simulink model "test_script"  (R2019b)
settings: Solver=VariableStepAuto  StartTime=0.0  StopTime=10.0  RelTol=1e-3
settings Model: Creator=FX622208  LastModifiedBy=FX622208

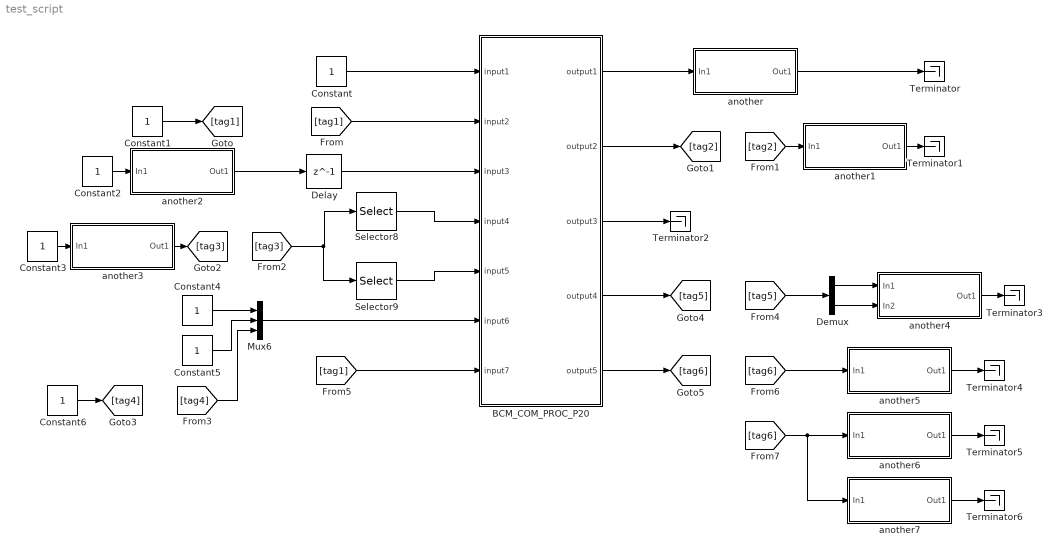
== system test_script ==
  BCM_COM_PROC_P20 : Subsystem
  Constant{,1..6} (7 alike) : Constant
  Delay : Delay  DelayLength=1  InitialCondition=0
  Demux : Demux  Outputs=2
  Mux6 : Mux  Inputs=3
  Selector8 : Selector  InputPortWidth=4  IndexOptions=Index vector (dialog)  Indices=[1 2]  OutputSizes=1
  Selector9 : Selector  InputPortWidth=4  IndexOptions=Index vector (dialog)  Indices=[3 4]  OutputSizes=1
  Terminator{,1..6} (7 alike) : Terminator
  another : Subsystem
  another1 : Subsystem
  another2 : Subsystem
  another3 : Subsystem
  another4 : Subsystem
  another5 : Subsystem
  another6 : Subsystem
  another7 : Subsystem
  wires:
  Constant/1 -> BCM_COM_PROC_P20/1(input1)
  BCM_COM_PROC_P20/1(output1) -> another/1(In1)
  [tag1] -> BCM_COM_PROC_P20/2(input2)
  Constant1/1 -> [tag1]
  BCM_COM_PROC_P20/2(output2) -> [tag2]
  [tag2] -> another1/1(In1)
  another/1(Out1) -> Terminator/1
  another1/1(Out1) -> Terminator1/1
  Constant2/1 -> another2/1(In1)
  another2/1(Out1) -> Delay/1
  Delay/1 -> BCM_COM_PROC_P20/3(input3)
  BCM_COM_PROC_P20/3(output3) -> Terminator2/1
  Selector8/1 -> BCM_COM_PROC_P20/4(input4)
  Selector9/1 -> BCM_COM_PROC_P20/5(input5)
  [tag3] -> Selector9/1, Selector8/1
  another3/1(Out1) -> [tag3]
  Constant3/1 -> another3/1(In1)
  Mux6/1 -> BCM_COM_PROC_P20/6(input6)
  Constant4/1 -> Mux6/1
  Constant5/1 -> Mux6/2
  [tag4] -> Mux6/3
  Constant6/1 -> [tag4]
  BCM_COM_PROC_P20/4(output4) -> [tag5]
  [tag5] -> Demux/1
  Demux/1 -> another4/1(In1)
  Demux/2 -> another4/2(In2)
  another4/1(Out1) -> Terminator3/1
  [tag1] -> BCM_COM_PROC_P20/7(input7)
  BCM_COM_PROC_P20/5(output5) -> [tag6]
  [tag6] -> another5/1(In1)
  another5/1(Out1) -> Terminator4/1
  another6/1(Out1) -> Terminator5/1
  [tag6] -> another7/1(In1), another6/1(In1)
  another7/1(Out1) -> Terminator6/1

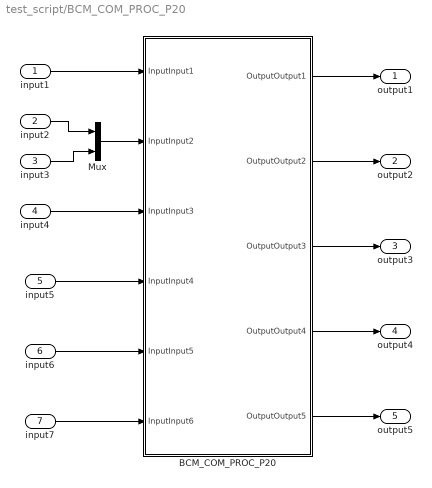
== system test_script/BCM_COM_PROC_P20 ==
  input1 : Inport
  input2 : Inport  Port=2
  input3 : Inport  Port=3
  input4 : Inport  Port=4
  input5 : Inport  Port=5
  input6 : Inport  Port=6
  input7 : Inport  Port=7
  BCM_COM_PROC_P20 : Subsystem
  Mux : Mux  Inputs=2
  output1 : Outport
  output2 : Outport  Port=2
  output3 : Outport  Port=3
  output4 : Outport  Port=4
  output5 : Outport  Port=5
  wires:
  input1/1 -> BCM_COM_PROC_P20/1(InputInput1)
  BCM_COM_PROC_P20/1(OutputOutput1) -> output1/1
  BCM_COM_PROC_P20/3(OutputOutput3) -> output3/1
  BCM_COM_PROC_P20/2(OutputOutput2) -> output2/1
  input2/1 -> Mux/1
  input3/1 -> Mux/2
  Mux/1 -> BCM_COM_PROC_P20/2(InputInput2)
  input4/1 -> BCM_COM_PROC_P20/3(InputInput3)
  BCM_COM_PROC_P20/4(OutputOutput4) -> output4/1
  input5/1 -> BCM_COM_PROC_P20/4(InputInput4)
  input6/1 -> BCM_COM_PROC_P20/5(InputInput5)
  input7/1 -> BCM_COM_PROC_P20/6(InputInput6)
  BCM_COM_PROC_P20/5(OutputOutput5) -> output5/1

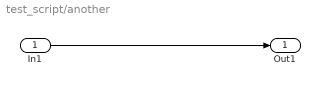
== system test_script/another ==
  In1 : Inport
  Out1 : Outport
  wires:
  In1/1 -> Out1/1

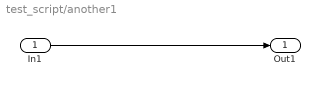
== system test_script/another1 ==
  In1 : Inport
  Out1 : Outport
  wires:
  In1/1 -> Out1/1

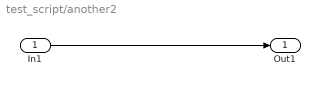
== system test_script/another2 ==
  In1 : Inport
  Out1 : Outport
  wires:
  In1/1 -> Out1/1

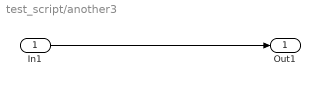
== system test_script/another3 ==
  In1 : Inport
  Out1 : Outport
  wires:
  In1/1 -> Out1/1

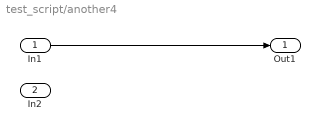
== system test_script/another4 ==
  In1 : Inport
  In2 : Inport  Port=2
  Out1 : Outport
  wires:
  In1/1 -> Out1/1

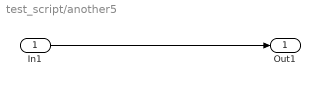
== system test_script/another5 ==
  In1 : Inport
  Out1 : Outport
  wires:
  In1/1 -> Out1/1

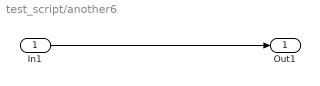
== system test_script/another6 ==
  In1 : Inport
  Out1 : Outport
  wires:
  In1/1 -> Out1/1

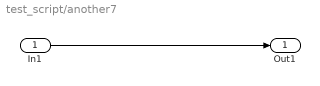
== system test_script/another7 ==
  In1 : Inport
  Out1 : Outport
  wires:
  In1/1 -> Out1/1

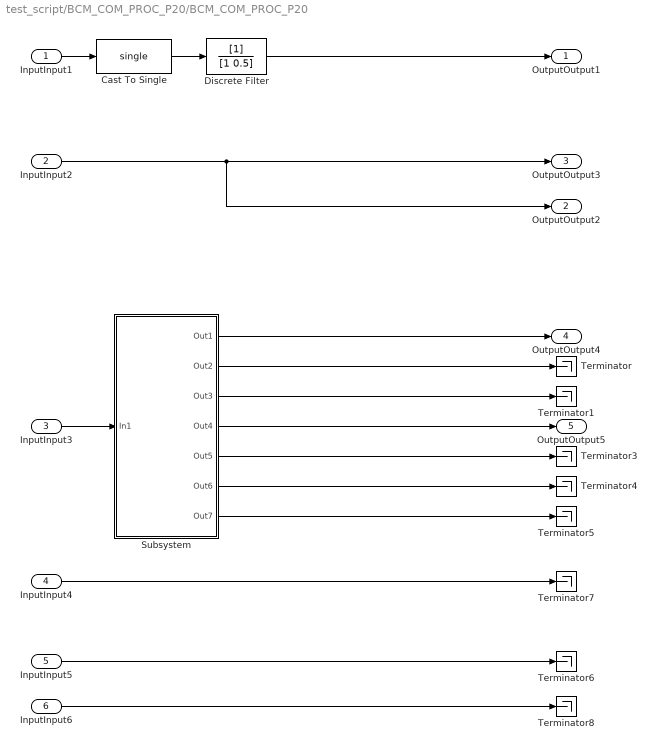
== system test_script/BCM_COM_PROC_P20/BCM_COM_PROC_P20 ==
  InputInput1 : Inport
  InputInput2 : Inport  Port=2
  InputInput3 : Inport  Port=3
  InputInput4 : Inport  Port=4
  InputInput5 : Inport  Port=5
  InputInput6 : Inport  Port=6
  Cast To Single : DataTypeConversion  OutDataTypeStr=single
  Discrete Filter : DiscreteFilter
  Subsystem : Subsystem
  Terminator{,1,3..8} (8 alike) : Terminator
  OutputOutput1 : Outport
  OutputOutput2 : Outport  Port=2
  OutputOutput3 : Outport  Port=3
  OutputOutput4 : Outport  Port=4
  OutputOutput5 : Outport  Port=5
  wires:
  InputInput1/1 -> Cast To Single/1
  Discrete Filter/1 -> OutputOutput1/1
  InputInput2/1 -> OutputOutput2/1, OutputOutput3/1
  InputInput3/1 -> Subsystem/1(In1)
  Subsystem/1(Out1) -> OutputOutput4/1
  Subsystem/2(Out2) -> Terminator/1
  Subsystem/3(Out3) -> Terminator1/1
  Subsystem/4(Out4) -> OutputOutput5/1
  Subsystem/5(Out5) -> Terminator3/1
  Subsystem/6(Out6) -> Terminator4/1
  Subsystem/7(Out7) -> Terminator5/1
  Cast To Single/1 -> Discrete Filter/1
  InputInput5/1 -> Terminator6/1
  InputInput4/1 -> Terminator7/1
  InputInput6/1 -> Terminator8/1

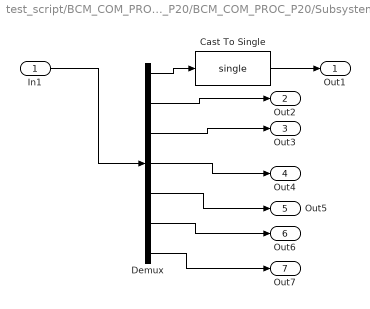
== system test_script/BCM_COM_PROC_P20/BCM_COM_PROC_P20/Subsystem ==
  In1 : Inport
  Cast To Single : DataTypeConversion  OutDataTypeStr=single
  Demux : Demux  Outputs=7
  Out1 : Outport
  Out2 : Outport  Port=2
  Out3 : Outport  Port=3
  Out4 : Outport  Port=4
  Out5 : Outport  Port=5
  Out6 : Outport  Port=6
  Out7 : Outport  Port=7
  wires:
  In1/1 -> Demux/1
  Demux/2 -> Out2/1
  Demux/3 -> Out3/1
  Demux/4 -> Out4/1
  Demux/5 -> Out5/1
  Demux/6 -> Out6/1
  Demux/7 -> Out7/1
  Cast To Single/1 -> Out1/1
  Demux/1 -> Cast To Single/1
